simulink model "TransientAnalysis"  (R2024a)
settings: Solver=ode23t  StartTime=0.0  StopTime=0.2  RelTol=1e-4
libraries: spsGroundLib x5, spsSeriesRLCBranchLib x4, spsACVoltageSourceLib x1, spsBreakerLib x1, spsVoltageMeasurementLib x1, spsCurrentMeasurementLib x1, spsParallelRLCLoadLib x1, spspowerguiLib x1
settings Model: Creator=The MathWorks, Inc.  LastModifiedBy=ayush
settings SolverCC: ZeroCrossAlgorithm=Adaptive  AlgebraicLoopSolver=TrustRegion
settings DataIOCC: SaveFormat=Array  ReturnWorkspaceOutputs=off  SignalLoggingName=sigsOut
settings OptimizationCC: BlockReduction=off  BooleanDataType=off  ExpressionDepthLimit=2147483647  InitFltsAndDblsToZero=on  EfficientMapNaN2IntZero=off  LifeSpan=inf
settings DebuggingCC: SaveWithParameterizedLinksMsg=none  UnderspecifiedInitializationDetection=Classic  MergeDetectMultiDrivingBlocksExec=none  CheckExecutionContextPreStartOutputMsg=on  SignalResolutionControl=TryResolveAllWithWarning  MultiTaskDSMMsg=warning  MultiTaskCondExecSysMsg=none  SigSpecEnsureSampleTimeMsg=none  FcnCallInpInsideContextMsg=warning  UnconnectedInputMsg=warning  UnconnectedOutputMsg=warning  UnconnectedLineMsg=warning  StateNameClashWarn=warning  SFUnexpectedBacktrackingDiag=warning  SFNoUnconditionalDefaultTransitionDiag=warning  SFExecutionAtInitializationDiag=none  ArithmeticOperatorsInVariantConditions=warning
settings HardwareCC: ProdBitPerPointer=32  ProdBitPerSizeT=32  ProdBitPerPtrDiffT=32  ProdLargestAtomicFloat=None  ProdIntDivRoundTo=Undefined  ProdEndianess=Unspecified  ProdWordSize=32  ProdHWDeviceType=32-bit Generic  TargetUnknown=on
settings ModelReferenceCC: EnableRefExpFcnMdlSchedulingChecks=on  PropagateSignalLabelsOutOfModel=off
settings SFSimCC: SimUseLocalCustomCode=off  CustomCodeUndefinedFunction=UseInterfaceOnly
settings RTWCC: RTWUseLocalCustomCode=off  GPUComputeCapability=3.5  DLArmComputeVersion=19.05
settings CodeAppCC: StateflowObjectComments=on
settings GRTTargetCC: TargetFcnLib=ansi_tfl_tmw.mat  TargetLangStandard=C89/C90 (ANSI)  CombineOutputUpdateFcns=off  GRTInterface=on
settings ConfigComp: CovMetricSettings=dw  CovSaveCumulativeToWorkspaceVar=on  CovSaveSingleToWorkspaceVar=on  CovExternalEMLEnable=off  CovSFcnEnable=off
settings SimscapeCC: SimscapeNormalizeSystem=off

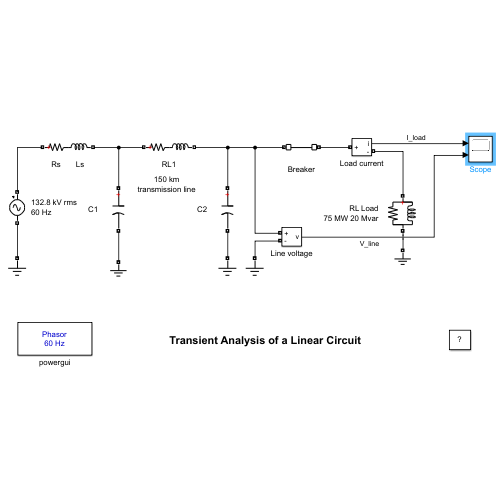
[thumbnail: Simulink's stored preview of the top-level diagram]
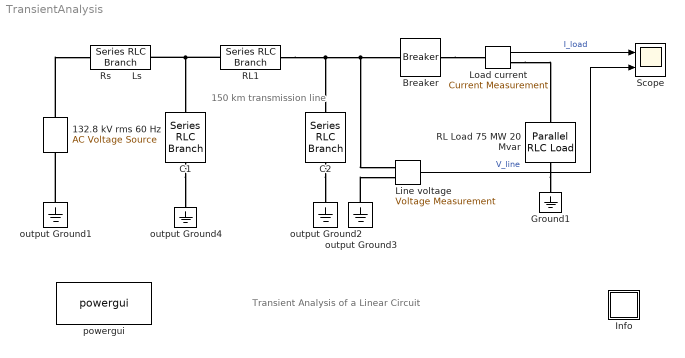
== system TransientAnalysis ==
  note: 150 km
      | transmission line
  note: Transient Analysis of a Linear Circuit
  132.8 kV rms 60 Hz : spsACVoltageSourceLib/AC Voltage Source  Description=source block  Amplitude=230e3/sqrt(3)*sqrt(2)  Phase=90  Frequency=60  SampleTime=0  Measurements=None  BusType=swing  Pref=10e3  Qref=0  Qmin=-inf  Qmax=+inf
      settings: AttributesFormatString=\n
  Breaker : spsBreakerLib/Breaker  InitialState=1  SwitchingTimes="[ 2/60  7/60 ]"  External=off  BreakerResistance=0.01  SnubberResistance=inf  SnubberCapacitance=0  Measurements=None  MoreParameters=off  NoBreakLoop=off
      settings: AttributesFormatString=\n
  C1 : spsSeriesRLCBranchLib/Series RLC Branch  LConnTagsString=__new0  RConnTagsString=__new0  BranchType=C  Resistance=[]  Inductance=[]  SetiL0=off  InitialCurrent=0  Capacitance=0.967e-06  Setx0=off  InitialVoltage=0  Measurements=None
  C2 : spsSeriesRLCBranchLib/Series RLC Branch  LConnTagsString=__new0  RConnTagsString=__new0  BranchType=C  Resistance=[]  Inductance=[]  SetiL0=off  InitialCurrent=0  Capacitance=0.967e-06  Setx0=off  InitialVoltage=0  Measurements=None
  Ground1 : spsGroundLib/Ground  LConnTagsString=a
  Info : Subsystem
      settings: OpenFcn="showExample(\"simscapeelectricalsps/TransientAnalysisExample\")"
      mask Display: disp('?')
  Line voltage : spsVoltageMeasurementLib/Voltage Measurement  Tag=PoWeRsYsTeMmEaSuReMeNt  PhasorSimulation=on  OutputType=Magnitude  PSBequivalent=0
  Load current : spsCurrentMeasurementLib/Current Measurement  Tag=PoWeRsYsTeMmEaSuReMeNt  PhasorSimulation=on  OutputType=Magnitude  PSBequivalent=0
      settings: AttributesFormatString=\n
  RL Load 75 MW 20 Mvar : spsParallelRLCLoadLib/Parallel RLC Load  LConnTagsString=a  RConnTagsString=__new0  NominalVoltage=132.8e3  NominalFrequency=60  ActivePower=75e6  InductivePower=20e6  CapacitivePower=0  Setx0=off  InitialVoltage=0  SetiL0=off  InitialCurrent=0  Measurements=None  LoadType=constant Z
      settings: AttributesFormatString=\n
  RL1 : spsSeriesRLCBranchLib/Series RLC Branch  LConnTagsString=__new0  RConnTagsString=__new0  BranchType=RL  Resistance=5.2  Inductance=138e-3  SetiL0=off  InitialCurrent=0  Capacitance=[]  Setx0=off  InitialVoltage=0  Measurements=None
  Rs       Ls : spsSeriesRLCBranchLib/Series RLC Branch  LConnTagsString=__new0  RConnTagsString=__new0  BranchType=RL  Resistance=2.645  Inductance=70.2e-03  SetiL0=off  InitialCurrent=0  Capacitance=[]  Setx0=off  InitialVoltage=0  Measurements=None
  Scope : Scope  NumInputPorts=2
  output Ground{1..4} (4 alike) : spsGroundLib/Ground  LConnTagsString=a
  powergui : spspowerguiLib/powergui  Priority=2  SimulationMode=Phasor  SampleTime=50e-6  frequency=60  Iterations=50  frequencyindice=60  Pbase=100e6  ErrMax=1e-4  UnitsV=kV  UnitsW=MW  buscounter=0  FunctionMessages=off  echomessages=off  EnableUseOfTLC=off  CurrentSourceSwitches=off  DisableSnubberDevices=on  DisableRonSwitches=off  DisableVfSwitches=off  DisplayEquations=off  AutomaticDiscreteSolvers=off  SolverType=Tustin  Interpol=off  ExternalGateDelay=off  methode=off  Ts=0  x0status=zero  SPID=on  SwTol=0  HookPort=off  NonlinearTolerance=1e-4  nMaxIteration=100  ContinueOnMaxIteration=off  RestoreLinks=warning  ResistiveCurrentMeasurement=off  Frange=logspace(0,3,50)  Ylog=off  Xlog=off  ShowGrid=off  save=off  variable=ZData  structure=0  ZoomFFT=on  StartTime=0.0  cycles=1  DisplayStyle=off  fundamental=60  FreqAxis=off  MaxFrequency=1000  frequencyindicesteady=1  RmsSteady=1  display=off
  wires:
  Line voltage/1 -> Scope/2  "V_line"
  Load current/1 -> Scope/1  "I_load"
  connections:
  RL Load 75 MW 20 Mvar/RConn1 -- Ground1/LConn1
  output Ground3/LConn1 -- Line voltage/LConn2
  RL1/RConn1 -- Line voltage/LConn1 -- Breaker/LConn1 -- C2/LConn1
  132.8 kV rms 60 Hz/RConn1 -- Rs       Ls/LConn1
  output Ground1/LConn1 -- 132.8 kV rms 60 Hz/LConn1
  Breaker/RConn1 -- Load current/LConn1
  Load current/RConn1 -- RL Load 75 MW 20 Mvar/LConn1
  RL1/LConn1 -- Rs       Ls/RConn1 -- C1/LConn1
  C1/RConn1 -- output Ground4/LConn1
  C2/RConn1 -- output Ground2/LConn1

== system TransientAnalysis/Info ==
